simulink model "test_PLLNoise"  (R2023b)
settings: Solver=VariableStepAuto  StartTime=0.0  StopTime=0.1  FixedStep=0.001  RelTol=1e-3
undefined symbols (not defined in the file): CN0, data
libraries: sensors_subsystems x1
settings Model: Creator=brent  LastModifiedBy=brent

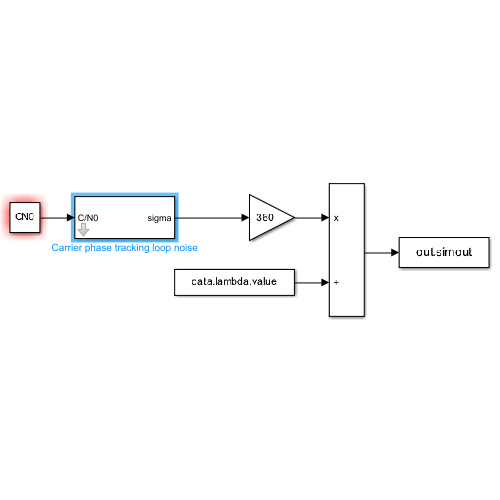
[thumbnail: Simulink's stored preview of the top-level diagram]
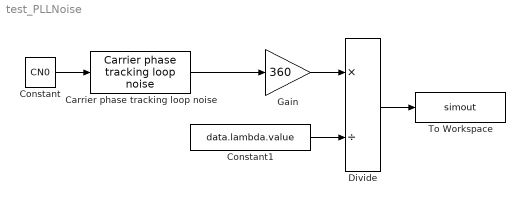
== system test_PLLNoise ==
  Carrier phase tracking loop noise : sensors_subsystems/Carrier phase tracking loop noise  Bn=data.Phase.Bn.value  T=data.Phase.T.value  lambda=data.lambda.value
      settings: SourceProductName=Sensors library
  Constant : Constant  Value=CN0
  Constant1 : Constant  Value=data.lambda.value
  Divide : Product  Inputs=*/
  Gain : Gain  Gain=360
  To Workspace : ToWorkspace  VariableName=simout  SaveFormat=Timeseries  SampleTime=-1
  wires:
  Constant/1 -> Carrier phase tracking loop noise/1
  Gain/1 -> Divide/1
  Constant1/1 -> Divide/2
  Divide/1 -> To Workspace/1
  Carrier phase tracking loop noise/1 -> Gain/1
